simulink model "testNetwork"  (R2013a)
settings: Solver=ode45  StartTime=0.0  StopTime=10.0  RelTol=1e-3
libraries: opticalComponentLibrary x6
settings Model: Creator=Nithya Menon  LastModifiedBy=Nithya Menon

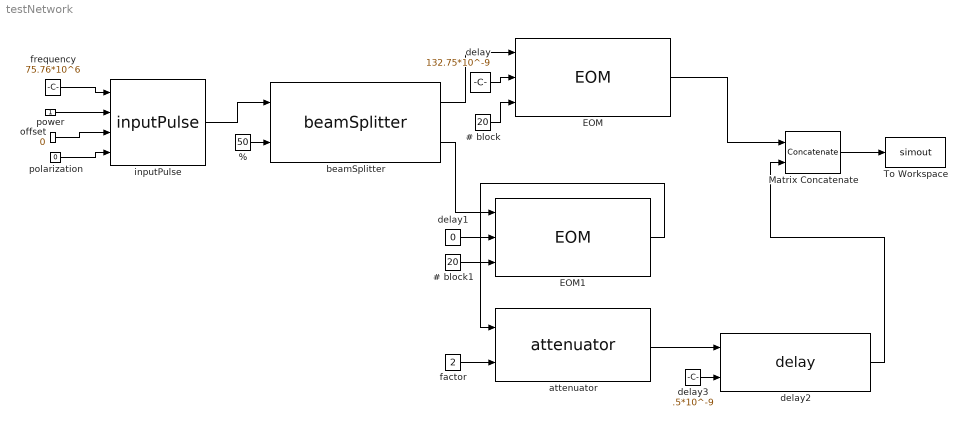
== system testNetwork ==
  # block : Constant  Value=20
  # block1 : Constant  Value=20
  % : Constant  Value=50
  EOM : opticalComponentLibrary/EOM
  EOM1 : opticalComponentLibrary/EOM
  Matrix Concatenate : Concatenate  Mode=Multidimensional array
  To Workspace : ToWorkspace  VariableName=simout  SampleTime=-1  SaveFormat=Timeseries
  attenuator : opticalComponentLibrary/attenuator
  beamSplitter : opticalComponentLibrary/beamSplitter
  delay : Constant  Value=132.75*10^-9
  delay1 : Constant  Value=0
  delay2 : opticalComponentLibrary/delay
  delay3 : Constant  Value=.5*10^-9
  factor : Constant  Value=2
  frequency : Constant  Value=75.76*10^6
  inputPulse : opticalComponentLibrary/inputPulse
  offset : Constant  Value=0
  polarization : Constant  Value=0
  power : Constant
  wires:
  polarization/1 -> inputPulse/4
  offset/1 -> inputPulse/3
  power/1 -> inputPulse/2
  frequency/1 -> inputPulse/1
  inputPulse/1 -> beamSplitter/1
  %/1 -> beamSplitter/2
  beamSplitter/1 -> EOM/1
  delay/1 -> EOM/2
  # block/1 -> EOM/3
  EOM/1 -> Matrix Concatenate/1
  beamSplitter/2 -> EOM1/1
  delay1/1 -> EOM1/2
  # block1/1 -> EOM1/3
  EOM1/1 -> attenuator/1
  factor/1 -> attenuator/2
  attenuator/1 -> delay2/1
  delay2/1 -> Matrix Concatenate/2
  delay3/1 -> delay2/2
  Matrix Concatenate/1 -> To Workspace/1
